simulink model "part2"  (R2024b)
settings: Solver=FixedStepAuto  StartTime=0.0  StopTime=0.05  FixedStep=1e-6  RelTol=1e-3
settings Model: Creator=Andrei  LastModifiedBy=Andrei

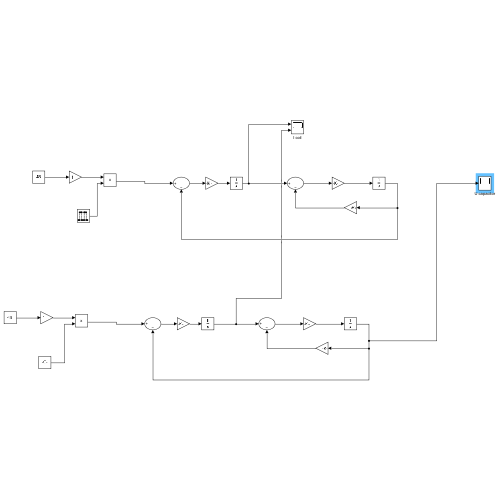
[thumbnail: Simulink's stored preview of the top-level diagram]
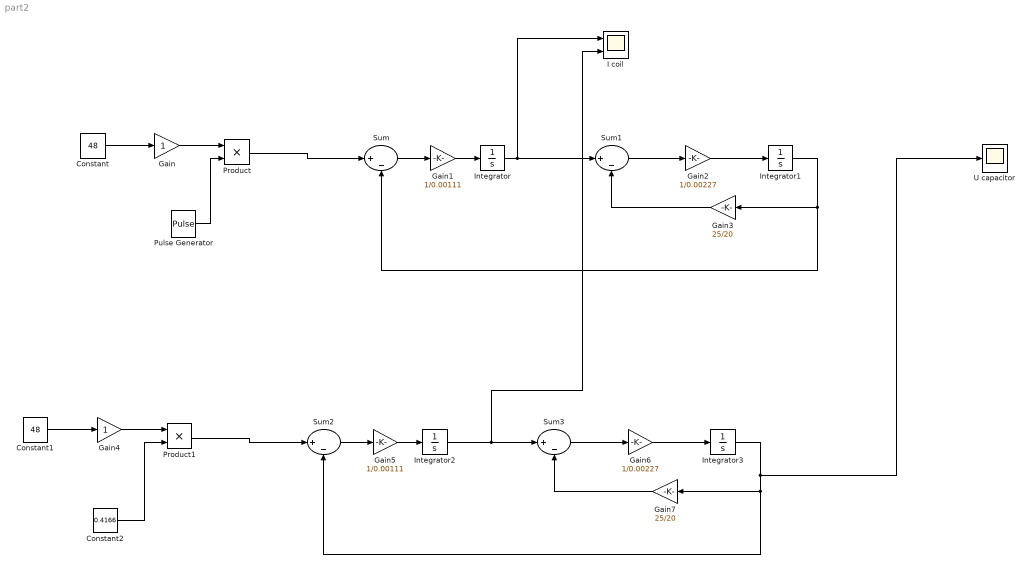
== system part2 ==
  Constant : Constant  Value=48
  Constant1 : Constant  Value=48
  Constant2 : Constant  Value=0.4166
  Gain : Gain
  Gain1 : Gain  Gain=1/0.00111
  Gain2 : Gain  Gain=1/0.00227
  Gain3 : Gain  Gain=25/20
  Gain4 : Gain
  Gain5 : Gain  Gain=1/0.00111
  Gain6 : Gain  Gain=1/0.00227
  Gain7 : Gain  Gain=25/20
  I coil : Scope  NumInputPorts=2
  Integrator{,1..3} (4 alike) : Integrator
  Product : Product
  Product1 : Product
  Pulse Generator : DiscretePulseGenerator  Period=1200  PulseWidth=504  SampleTime=1e-6
  Sum{,1..3} (4 alike) : Sum  Inputs=|+-
  U capacitor : Scope
  wires:
  Product/1 -> Sum/1
  Pulse Generator/1 -> Product/2
  Constant/1 -> Gain/1
  Gain/1 -> Product/1
  Sum/1 -> Gain1/1
  Gain1/1 -> Integrator/1
  Integrator1/1 -> Gain3/1, Sum/2
  Sum1/1 -> Gain2/1
  Gain2/1 -> Integrator1/1
  Gain3/1 -> Sum1/2
  Integrator/1 -> I coil/1, Sum1/1
  Integrator3/1 -> U capacitor/1, Gain7/1, Sum2/2
  Constant1/1 -> Gain4/1
  Gain6/1 -> Integrator3/1
  Gain7/1 -> Sum3/2
  Product1/1 -> Sum2/1
  Sum3/1 -> Gain6/1
  Gain4/1 -> Product1/1
  Gain5/1 -> Integrator2/1
  Integrator2/1 -> I coil/2, Sum3/1
  Sum2/1 -> Gain5/1
  Constant2/1 -> Product1/2
